simulink model "Gesamtsystem_Prototyp25_01_3"  (R2021b)
settings: Solver=FixedStepDiscrete  StartTime=0.0  StopTime=Inf  RelTol=1e-3  EnableMultiTasking=on
undefined symbols (not defined in the file): Down, GPTRIP1SEL, GPTRIP2SEL, magnitude, TZ1, TZ2, Up
libraries: c2837xDlib x18, hdlsllib x10, simulink x5, c2802xlib x5, c280xlib x3, dspsigops x3, commsequence2 x2, idelinklib_common x2, mcbcontrolslib x2, c2000lib x1, dspstat3 x1
(part 2 of 3)

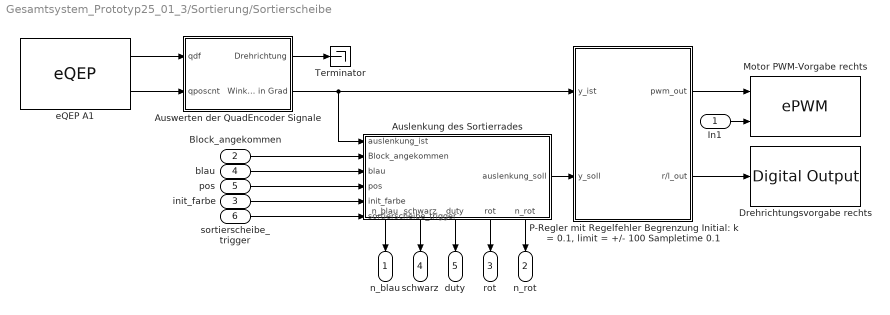
== system Gesamtsystem_Prototyp25_01_3/Sortierung/Sortierscheibe ==
  In1 : Inport
  Block_angekommen : Inport  Port=2
  init_farbe : Inport  Port=3
  blau : Inport  Port=4
  pos : Inport  Port=5
  sortierscheibe_trigger : Inport  Port=6
  Auslenkung des Sortierrades : Stateflow chart  TreatAsAtomicUnit=on
      settings: PortSchema="{\"entries\":[{\"content\":{\"sides\":[{\"content\":{\"connectorIds\":[\"In3\",\"In2\",\"In4\",\"In5\",\"In6\",\"In1\"]},\"type\":\"ConnectorPlacement.EquallySpacedRectSide\",\"uuid\":\"50e19062-f064-4bab-8c9d-33b65ef4a937\"},{\"content\":{\"connectorIds\":[\"Out5\"],\"side\":\"RIGHT\"},\"type\":\"ConnectorPlacement.EquallySpacedRectSide\",\"uuid\":\"30a7e15c-c340-43b9-b3db-9e571d923d3f\"},{\"content\":{\"connectorIds\":[],\"side\":\"TOP\"},\"type\":\"ConnectorPlacement.EquallySpacedRectSide\",\"uuid\":\"40fbcefe-2254-4087-9ee2-3aa6f0d07988\"},{\"content\":{\"connectorIds\":[\"Out4\",\"Out6\",\"Out2\",\"Out3\",\"Out1\"],\"side\":\"BOTTOM\"},\"type\":\"ConnectorPlacement.EquallySpacedRectSide\",\"uuid\":\"44f37ab7-e4d3-4b33-8443-86555161b992\"}]},\"type\":\"ConnectorPlacement.EquallySpacedConnector\",\"uuid\":\"9a2bc586-2b2b-4dda-85c2-1e199ea03007\"}],\"packageUris\":[\"http://schema.mathworks.com/mf0/Connector/R2020b\"],\"version\":\"1.0\"}"
  Auswerten der QuadEncoder Signale : Subsystem
  Drehrichtungsvorgabe rechts : c2837xDlib/Digital Output  GPIO_Number=GPIO88~GPIO95  GPIO_Bit0=off  GPIO_BIT0_Toggle=off  GPIO_Bit1=off  GPIO_BIT1_Toggle=off  GPIO_Bit2=off  GPIO_BIT2_Toggle=off  GPIO_Bit3=off  GPIO_BIT3_Toggle=off  GPIO_Bit4=off  GPIO_BIT4_Toggle=off  GPIO_Bit5=off  GPIO_BIT5_Toggle=off  GPIO_Bit6=on  GPIO_BIT6_Toggle=off  GPIO_Bit7=off  GPIO_BIT7_Toggle=off
      settings: SourceProductBaseCode=TIC2000
  Motor PWM-Vorgabe rechts : c2802xlib/ePWM  PwmType=C2000_Type4  useModule=ePWM6  ePWMxLINKTBPRD=Not Linked  periodUnits=Clock cycles  timerSource=Specify via dialog  timerPeriod_clk=64000  timerPeriod_sec=0.0001  tbshadow=Counter equals to zero  countingMode=Up-Down  phaseActiveEnable=Disable  phaseDirection=Count down after sync  phaseActive=0  synchronizationEnable=off  dcaevt1Sync=off  dcbevt1Sync=off  synchronizationOption=Disable  perSynchronizationOption=Counter equals to period (CTR=PRD)  clockPrescale=1  HSclockPrescale=1  enswap=off  ePWMxAStatus=on  ePWMxAactionLogic1=Set  ePWMxAactionLogic2=Clear  ePWMxAactionLogic3=Clear  ePWMxAactionLogic4=Set  ePWMxAactionLogic5=Do nothing  ePWMxAactionLogic6=Do nothing  ePWMxACSFenable=off  ePWMxACSFvalue=Forcing disable  ePWMxASFreload=Zero  ePWMxBStatus=on  ePWMxBactionLogic1=Set  ePWMxBactionLogic2=Clear  ePWMxBactionLogic3=Do nothing  ePWMxBactionLogic4=Do nothing  ePWMxBactionLogic5=Clear  ePWMxBactionLogic6=Set  ePWMxBCSFenable=off  ePWMxBCSFvalue=Forcing disable  ePWMxBSFreload=Zero  ePWNxBOutWay=off  ePWMxLINKCMPA=Not Linked  CMPAUnits=Percentages  CMPASource=Input port  CMPAValue_per=50  CMPAValue_clk=32000  enCMPAshadow=Counter equals to zero (CTR=Zero)  ePWMxLINKCMPB=Not Linked  CMPBUnits=Percentages  CMPBSource=Input port  CMPBValue_per=25  CMPBValue_clk=32000  enCMPBshadow=Counter equals to zero (CTR=Zero)  ePWMxLINKCMPC=Not Linked  CMPCUnits=Clock cycles  CMPCSource=Specify via dialog  CMPCValue_per=50  CMPCValue_clk=32000  enCMPCshadow=Counter equals to zero (CTR=Zero)  ePWMxLINKCMPD=Not Linked  CMPDUnits=Clock cycles  CMPDSource=Specify via dialog  CMPDValue_per=50  CMPDValue_clk=32000  enCMPDshadow=Counter equals to zero (CTR=Zero)  enableDBePWMxA=off  enableDBePWMxB=off  enhalfcycle=off  DBpolarity=Active high (AH)  DBedgeDelay=Positive  DBSource_ePWMxA=ePWMxA  DBSource_ePWMxB=ePWMxA  DBPeriodUnits=Clock cycles  DBperiodSource=Specify via dialog  REDperiod=0  FEDperiod=0  REDperiod_sec=0  FEDperiod_sec=0  LoadModeDBRED=Immediate without using shadow  LoadModeDBFED=Immediate without using shadow  adcstartModuleA=off  adcrequestEventA=First event  adcstartEventA=Digital Compare Module A Event 1 start of conversion (DCAEVT1.soc)  adcstartEventA_type2=Digital Compare Module A Event 1 start of conversion (DCAEVT1.soc)  adcstartModuleB=off  adcrequestEventB=First event  adcstartEventB=Counter equals to zero (CTR=Zero)  adcstartEventB_type2=Counter equals to zero (CTR=Zero)  intEn=off  intPrd=First event  intSel=Counter equals to zero (CTR=Zero)  intSel_type2=Counter equals to zero (CTR=Zero)  hrpe=off  enHRPWM=off  HRPWM_LoadMode=Counter equals to period (CTR=PRD)  HRPWM_CTLMode=Duty or Period control mode  HRPWM_EDGMode=Both edge  hrpeb=off  enHRPWMB=off  HRPWM_LoadModeB=Counter equals to zero (CTR=ZERO)  HRPWM_CTLModeB=Duty or Period control mode  HRPWM_EDGModeB=Both edge  enHRDBRED=off  enHRDBFED=off  enSFO=on  enautoconv=on  chopperEnable=off  chopperFrequency=1  chopperFirstwidth=1  chopperDuty=12.5%  tripZonesource=Specify via dialog  tzselOSHT1=off  tzselOSHT2=off  tzselOSHT3=off  tzselOSHDCAEV1=off  tzselOSHDCBEV1=off  tzselCBC1=off  tzselCBC2=off  tzselCBC3=off  tzselCBCDCAEV2=off  tzselCBCDCBEV2=off  tzselOSHT4=off  tzselOSHT5=off  tzselOSHT6=off  tzselCBC4=off  tzselCBC5=off  tzselCBC6=off  enTzOstIntr=off  enTzCbcIntr=off  enTzDCAEVT1Intr=off  enTzDCAEVT2Intr=off  enTzDCBEVT1Intr=off  enTzDCBEVT2Intr=off  ePWMxAforced=No action  ePWMxBforced=No action  DCAEVT1forced=No action  DCBEVT1forced=No action  DCAEVT2forced=No action  DCBEVT2forced=No action  dcah=Trip Zone 1 input (TZ1)  dcal=Trip Zone 2 input (TZ2)  dcbh=Trip Zone 1 input (TZ1)  dcbl=Trip Zone 2 input (TZ2)  dcah_type2=GPTRIP1SEL/(TZ1)  dcal_type2=GPTRIP2SEL/(TZ2)  dcbh_type2=GPTRIP1SEL/(TZ1)  dcbl_type2=GPTRIP2SEL/(TZ2)  gendcaevt1=Event disabled  gendcaevt2=Event disabled  gendcbevt1=Event disabled  gendcbevt2=Event disabled  dcaevt1src=DCAEVT1 with sync  dcaevt2src=DCAEVT2 with sync  dcbevt1src=DCBEVT1 with sync  dcbevt2src=DCBEVT2 with sync  pulsesel=Counter equals to zero (CTR=Zero)  blankinv=off  blankoffset=0  blankwidth=0  evsrcsel=Filtered version of DCAEVT1 (DCAEVT1FILT)  encape=off
  "P-Regler mit Regelfehler Begrenzung Initial: k = 0.1, limit = +/- 100 Sampletime 0.1" : Subsystem
  Terminator : Terminator
  eQEP A1 : c280xlib/eQEP  useModule=eQEP1  pcInputmode=Quadrature-count  externalClockrate=2x resolution: Count the rising/falling edge  swapPolarityselection=Clockwise  qdfOutputport=on  qapPolarityselection=off  qbpPolarityselection=off  qipPolarityselection=off  qspPolarityselection=off  igatePolarityselection=off  sampleTime=0.01  pcOutputport=on  pcMaximumvalue=4294967295  indexInitializationcheck=off  indexInitializationevent=Rising edge  strobeInitializationcheck=off  strobeInitializationevent=Rising edge  softwareInitializationcheck=off  softwareInitializationsource=Set to init value at start up  softwareInitializationmode=on  pcInitialvalue=2147483648  pcResetmode=Reset on an index event  ieloutputport=off  indexEventlatch=Rising edge  seloutputport=off  strobeEventlatch=Rising edge  pcefOutputport=off  enableEqepcapture=off  qctmrOutputport=off  qcprdOutputport=off  captureTimerprescaler=128  upEventprescaler=128  overflowErrorflag=off  directionErrorflag=off  captureTimerposition=On position counter read  unitTimerperiod=100000000  captureTimerlatch=off  capturePeriodlatch=off  positionCounterlatch=off  soenPolarityselection=off  spselPolarityselection=Index pin is used for sync output  compareValuesource=Specify via dialog  shadowMode=Load on QPOSCNT=0  compareValue=4294967295  syncOutputwidth=1  polaritySyncoutput=Active high  watchdogEnable=off  watchdogTimer=65535  outport1Datatype=auto  outport2Datatype=auto  outport3Datatype=auto  outport4Datatype=auto  outport5Datatype=auto  outport6Datatype=auto  outport7Datatype=auto  outport8Datatype=auto  outport9Datatype=auto  outport10Datatype=auto  outport11Datatype=auto  outport12Datatype=auto  eqepinterrupt_pce=off  eqepinterrupt_qpe=off  eqepinterrupt_qdc=off  eqepinterrupt_wto=off  eqepinterrupt_pcu=off  eqepinterrupt_pco=off  eqepinterrupt_pcr=off  eqepinterrupt_pcm=off  eqepinterrupt_sel=off  eqepinterrupt_iel=off  eqepinterrupt_uto=off  pheOutputport=off  watchdogOutputport=off  outport13Datatype=auto  outport14Datatype=auto
      settings: SourceProductBaseCode=TIC2000
  n_blau : Outport
  n_rot : Outport  Port=2
  rot : Outport  Port=3
  schwarz : Outport  Port=4
  duty : Outport  Port=5
  wires:
  In1/1 -> Motor PWM-Vorgabe rechts/2
  eQEP A1/1 -> Auswerten der QuadEncoder Signale/1(qdf)
  Auslenkung des Sortierrades/5(auslenkung_soll) -> "P-Regler mit Regelfehler Begrenzung Initial: k = 0.1, limit = +/- 100 Sampletime 0.1"/2(y_soll)
  "P-Regler mit Regelfehler Begrenzung Initial: k = 0.1, limit = +/- 100 Sampletime 0.1"/2(r/l_out) -> Drehrichtungsvorgabe rechts/1
  "P-Regler mit Regelfehler Begrenzung Initial: k = 0.1, limit = +/- 100 Sampletime 0.1"/1(pwm_out) -> Motor PWM-Vorgabe rechts/1
  Auswerten der QuadEncoder Signale/2(Winkel in Grad) -> Auslenkung des Sortierrades/3(auslenkung_ist), "P-Regler mit Regelfehler Begrenzung Initial: k = 0.1, limit = +/- 100 Sampletime 0.1"/1(y_ist)
  eQEP A1/2 -> Auswerten der QuadEncoder Signale/2(qposcnt)
  blau/1 -> Auslenkung des Sortierrades/4(blau)
  Block_angekommen/1 -> Auslenkung des Sortierrades/2(Block_angekommen)
  pos/1 -> Auslenkung des Sortierrades/5(pos)
  Auswerten der QuadEncoder Signale/1(Drehrichtung) -> Terminator/1
  Auslenkung des Sortierrades/1(n_rot) -> n_rot/1
  Auslenkung des Sortierrades/4(n_blau) -> n_blau/1
  Auslenkung des Sortierrades/3(rot) -> rot/1
  Auslenkung des Sortierrades/6(schwarz) -> schwarz/1
  Auslenkung des Sortierrades/2(duty) -> duty/1
  init_farbe/1 -> Auslenkung des Sortierrades/6(init_farbe)
  sortierscheibe_trigger/1 -> Auslenkung des Sortierrades/1(sortierscheibe_trigger)

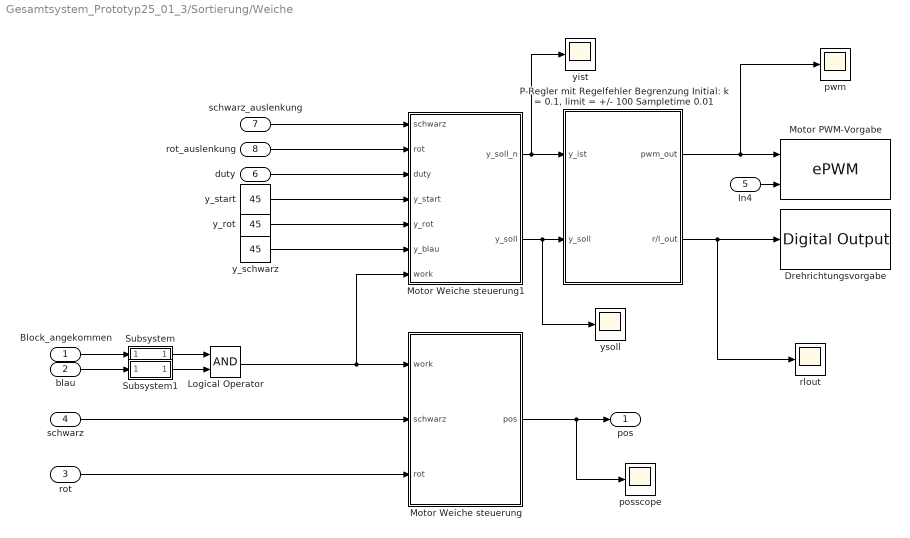
== system Gesamtsystem_Prototyp25_01_3/Sortierung/Weiche ==
  Block_angekommen : Inport
  blau : Inport  Port=2
  rot : Inport  Port=3
  schwarz : Inport  Port=4
  In4 : Inport  Port=5
  duty : Inport  Port=6
  schwarz_auslenkung : Inport  Port=7
  rot_auslenkung : Inport  Port=8
  Drehrichtungsvorgabe : c2837xDlib/Digital Output  GPIO_Number=GPIO120~GPIO127  GPIO_Bit0=off  GPIO_BIT0_Toggle=off  GPIO_Bit1=off  GPIO_BIT1_Toggle=off  GPIO_Bit2=off  GPIO_BIT2_Toggle=off  GPIO_Bit3=on  GPIO_BIT3_Toggle=off  GPIO_Bit4=off  GPIO_BIT4_Toggle=off  GPIO_Bit5=off  GPIO_BIT5_Toggle=off  GPIO_Bit6=off  GPIO_BIT6_Toggle=off  GPIO_Bit7=off  GPIO_BIT7_Toggle=off
      settings: SourceProductBaseCode=TIC2000
  Logical Operator : Logic  AllPortsSameDT=off  OutDataTypeStr=boolean
  Motor PWM-Vorgabe : c2802xlib/ePWM  PwmType=C2000_Type4  useModule=ePWM1  ePWMxLINKTBPRD=Not Linked  periodUnits=Clock cycles  timerSource=Specify via dialog  timerPeriod_clk=64000  timerPeriod_sec=0.0001  tbshadow=Counter equals to zero  countingMode=Up-Down  phaseActiveEnable=Disable  phaseDirection=Count down after sync  phaseActive=0  synchronizationEnable=off  dcaevt1Sync=off  dcbevt1Sync=off  synchronizationOption=Disable  perSynchronizationOption=Counter equals to period (CTR=PRD)  clockPrescale=1  HSclockPrescale=1  enswap=off  ePWMxAStatus=on  ePWMxAactionLogic1=Set  ePWMxAactionLogic2=Clear  ePWMxAactionLogic3=Clear  ePWMxAactionLogic4=Set  ePWMxAactionLogic5=Do nothing  ePWMxAactionLogic6=Do nothing  ePWMxACSFenable=off  ePWMxACSFvalue=Forcing disable  ePWMxASFreload=Zero  ePWMxBStatus=on  ePWMxBactionLogic1=Set  ePWMxBactionLogic2=Clear  ePWMxBactionLogic3=Do nothing  ePWMxBactionLogic4=Do nothing  ePWMxBactionLogic5=Clear  ePWMxBactionLogic6=Set  ePWMxBCSFenable=off  ePWMxBCSFvalue=Forcing disable  ePWMxBSFreload=Zero  ePWNxBOutWay=off  ePWMxLINKCMPA=Not Linked  CMPAUnits=Percentages  CMPASource=Input port  CMPAValue_per=50  CMPAValue_clk=32000  enCMPAshadow=Counter equals to zero (CTR=Zero)  ePWMxLINKCMPB=Not Linked  CMPBUnits=Percentages  CMPBSource=Input port  CMPBValue_per=25  CMPBValue_clk=32000  enCMPBshadow=Counter equals to zero (CTR=Zero)  ePWMxLINKCMPC=Not Linked  CMPCUnits=Clock cycles  CMPCSource=Specify via dialog  CMPCValue_per=50  CMPCValue_clk=32000  enCMPCshadow=Counter equals to zero (CTR=Zero)  ePWMxLINKCMPD=Not Linked  CMPDUnits=Clock cycles  CMPDSource=Specify via dialog  CMPDValue_per=50  CMPDValue_clk=32000  enCMPDshadow=Counter equals to zero (CTR=Zero)  enableDBePWMxA=off  enableDBePWMxB=off  enhalfcycle=off  DBpolarity=Active high (AH)  DBedgeDelay=Positive  DBSource_ePWMxA=ePWMxA  DBSource_ePWMxB=ePWMxA  DBPeriodUnits=Clock cycles  DBperiodSource=Specify via dialog  REDperiod=0  FEDperiod=0  REDperiod_sec=0  FEDperiod_sec=0  LoadModeDBRED=Immediate without using shadow  LoadModeDBFED=Immediate without using shadow  adcstartModuleA=off  adcrequestEventA=First event  adcstartEventA=Digital Compare Module A Event 1 start of conversion (DCAEVT1.soc)  adcstartEventA_type2=Digital Compare Module A Event 1 start of conversion (DCAEVT1.soc)  adcstartModuleB=off  adcrequestEventB=First event  adcstartEventB=Counter equals to zero (CTR=Zero)  adcstartEventB_type2=Counter equals to zero (CTR=Zero)  intEn=off  intPrd=First event  intSel=Counter equals to zero (CTR=Zero)  intSel_type2=Counter equals to zero (CTR=Zero)  hrpe=off  enHRPWM=off  HRPWM_LoadMode=Counter equals to period (CTR=PRD)  HRPWM_CTLMode=Duty or Period control mode  HRPWM_EDGMode=Both edge  hrpeb=off  enHRPWMB=off  HRPWM_LoadModeB=Counter equals to zero (CTR=ZERO)  HRPWM_CTLModeB=Duty or Period control mode  HRPWM_EDGModeB=Both edge  enHRDBRED=off  enHRDBFED=off  enSFO=on  enautoconv=on  chopperEnable=off  chopperFrequency=1  chopperFirstwidth=1  chopperDuty=12.5%  tripZonesource=Specify via dialog  tzselOSHT1=off  tzselOSHT2=off  tzselOSHT3=off  tzselOSHDCAEV1=off  tzselOSHDCBEV1=off  tzselCBC1=off  tzselCBC2=off  tzselCBC3=off  tzselCBCDCAEV2=off  tzselCBCDCBEV2=off  tzselOSHT4=off  tzselOSHT5=off  tzselOSHT6=off  tzselCBC4=off  tzselCBC5=off  tzselCBC6=off  enTzOstIntr=off  enTzCbcIntr=off  enTzDCAEVT1Intr=off  enTzDCAEVT2Intr=off  enTzDCBEVT1Intr=off  enTzDCBEVT2Intr=off  ePWMxAforced=No action  ePWMxBforced=No action  DCAEVT1forced=No action  DCBEVT1forced=No action  DCAEVT2forced=No action  DCBEVT2forced=No action  dcah=Trip Zone 1 input (TZ1)  dcal=Trip Zone 2 input (TZ2)  dcbh=Trip Zone 1 input (TZ1)  dcbl=Trip Zone 2 input (TZ2)  dcah_type2=GPTRIP1SEL/(TZ1)  dcal_type2=GPTRIP2SEL/(TZ2)  dcbh_type2=GPTRIP1SEL/(TZ1)  dcbl_type2=GPTRIP2SEL/(TZ2)  gendcaevt1=Event disabled  gendcaevt2=Event disabled  gendcbevt1=Event disabled  gendcbevt2=Event disabled  dcaevt1src=DCAEVT1 with sync  dcaevt2src=DCAEVT2 with sync  dcbevt1src=DCBEVT1 with sync  dcbevt2src=DCBEVT2 with sync  pulsesel=Counter equals to zero (CTR=Zero)  blankinv=off  blankoffset=0  blankwidth=0  evsrcsel=Filtered version of DCAEVT1 (DCAEVT1FILT)  encape=off
  Motor Weiche steuerung : Stateflow chart  TreatAsAtomicUnit=on
      settings: PortSchema="{\"entries\":[{\"content\":{\"sides\":[{\"content\":{\"connectorIds\":[\"In3\",\"In2\",\"In1\"]},\"type\":\"ConnectorPlacement.EquallySpacedRectSide\",\"uuid\":\"171d8009-52fc-4483-b4bb-3a0c0e7f0866\"},{\"content\":{\"connectorIds\":[\"Out1\"],\"side\":\"RIGHT\"},\"type\":\"ConnectorPlacement.EquallySpacedRectSide\",\"uuid\":\"a1e5e039-26f6-455c-94ae-620f09ecad1d\"},{\"content\":{\"connectorIds\":[],\"side\":\"TOP\"},\"type\":\"ConnectorPlacement.EquallySpacedRectSide\",\"uuid\":\"92e8292a-84f4-4654-b9a0-01a34f9604a2\"}]},\"type\":\"ConnectorPlacement.EquallySpacedConnector\",\"uuid\":\"f344f6ae-6777-4ef0-95d5-423a355c19db\"}],\"packageUris\":[\"http://schema.mathworks.com/mf0/Connector/R2020b\"],\"version\":\"1.0\"}"
  Motor Weiche steuerung1 : Stateflow chart  TreatAsAtomicUnit=on
      settings: PortSchema="{\"entries\":[{\"content\":{\"sides\":[{\"content\":{\"connectorIds\":[\"In2\",\"In1\",\"In7\",\"In4\",\"In5\",\"In6\",\"In3\"]},\"type\":\"ConnectorPlacement.EquallySpacedRectSide\",\"uuid\":\"171d8009-52fc-4483-b4bb-3a0c0e7f0866\"},{\"content\":{\"connectorIds\":[\"Out1\",\"Out2\"],\"side\":\"RIGHT\"},\"type\":\"ConnectorPlacement.EquallySpacedRectSide\",\"uuid\":\"a1e5e039-26f6-455c-94ae-620f09ecad1d\"},{\"content\":{\"connectorIds\":[],\"side\":\"TOP\"},\"type\":\"ConnectorPlacement.EquallySpacedRectSide\",\"uuid\":\"92e8292a-84f4-4654-b9a0-01a34f9604a2\"}]},\"type\":\"ConnectorPlacement.EquallySpacedConnector\",\"uuid\":\"f344f6ae-6777-4ef0-95d5-423a355c19db\"}],\"packageUris\":[\"http://schema.mathworks.com/mf0/Connector/R2020b\"],\"version\":\"1.0\"}"
  "P-Regler mit Regelfehler Begrenzung Initial: k = 0.1, limit = +/- 100 Sampletime 0.01" : Subsystem
  Subsystem : Subsystem
  Subsystem1 : Subsystem
  posscope : Scope
  pwm : Scope
  rlout : Scope
  y_rot : Constant  Value=45
  y_schwarz : Constant  Value=45
  y_start : Constant  Value=45
  yist : Scope
  ysoll : Scope
  pos : Outport
  wires:
  In4/1 -> Motor PWM-Vorgabe/2
  Subsystem1/1(Out1) -> Logical Operator/2
  Subsystem/1(Out1) -> Logical Operator/1
  Logical Operator/1 -> Motor Weiche steuerung1/3(work), Motor Weiche steuerung/3(work)
  rot/1 -> Motor Weiche steuerung/1(rot)
  Motor Weiche steuerung1/1(y_soll_n) -> "P-Regler mit Regelfehler Begrenzung Initial: k = 0.1, limit = +/- 100 Sampletime 0.01"/1(y_ist), yist/1
  Motor Weiche steuerung1/2(y_soll) -> ysoll/1, "P-Regler mit Regelfehler Begrenzung Initial: k = 0.1, limit = +/- 100 Sampletime 0.01"/2(y_soll)
  Block_angekommen/1 -> Subsystem/1(In1)
  "P-Regler mit Regelfehler Begrenzung Initial: k = 0.1, limit = +/- 100 Sampletime 0.01"/1(pwm_out) -> pwm/1, Motor PWM-Vorgabe/1
  "P-Regler mit Regelfehler Begrenzung Initial: k = 0.1, limit = +/- 100 Sampletime 0.01"/2(r/l_out) -> rlout/1, Drehrichtungsvorgabe/1
  blau/1 -> Subsystem1/1(In1)
  Motor Weiche steuerung/1(pos) -> posscope/1, pos/1
  y_start/1 -> Motor Weiche steuerung1/4(y_start)
  y_rot/1 -> Motor Weiche steuerung1/5(y_rot)
  y_schwarz/1 -> Motor Weiche steuerung1/6(y_blau)
  rot_auslenkung/1 -> Motor Weiche steuerung1/1(rot)
  duty/1 -> Motor Weiche steuerung1/7(duty)
  schwarz_auslenkung/1 -> Motor Weiche steuerung1/2(schwarz)
  schwarz/1 -> Motor Weiche steuerung/2(schwarz)

== system Gesamtsystem_Prototyp25_01_3/Sortierung/trigger initialisierung farbe ==
  Digital Input : c2837xDlib/Digital Input  GPIO_Number=GPIO0~GPIO7  GPIO_Bit0=off  GPIO_Bit1=off  GPIO_Bit2=off  GPIO_Bit3=on  GPIO_Bit4=off  GPIO_Bit5=off  GPIO_Bit6=off  GPIO_Bit7=off  sampleTime=0.1  dataType=auto  GPIO_Bit0_Qualification=Sync to SYSCLKOUT  GPIO_Bit1_Qualification=Sync to SYSCLKOUT  GPIO_Bit2_Qualification=Sync to SYSCLKOUT  GPIO_Bit3_Qualification=Sync to SYSCLKOUT  GPIO_Bit4_Qualification=Sync to SYSCLKOUT  GPIO_Bit5_Qualification=Sync to SYSCLKOUT  GPIO_Bit6_Qualification=Sync to SYSCLKOUT  GPIO_Bit7_Qualification=Sync to SYSCLKOUT  Qualification_Period=-1
      settings: SourceProductBaseCode=TIC2000
  Digital Input1 : c2837xDlib/Digital Input  GPIO_Number=GPIO0~GPIO7  GPIO_Bit0=off  GPIO_Bit1=off  GPIO_Bit2=off  GPIO_Bit3=off  GPIO_Bit4=on  GPIO_Bit5=off  GPIO_Bit6=off  GPIO_Bit7=off  sampleTime=0.1  dataType=auto  GPIO_Bit0_Qualification=Sync to SYSCLKOUT  GPIO_Bit1_Qualification=Sync to SYSCLKOUT  GPIO_Bit2_Qualification=Sync to SYSCLKOUT  GPIO_Bit3_Qualification=Sync to SYSCLKOUT  GPIO_Bit4_Qualification=Sync to SYSCLKOUT  GPIO_Bit5_Qualification=Sync to SYSCLKOUT  GPIO_Bit6_Qualification=Sync to SYSCLKOUT  GPIO_Bit7_Qualification=Sync to SYSCLKOUT  Qualification_Period=-1
      settings: SourceProductBaseCode=TIC2000
  Logical Operator : Logic  AllPortsSameDT=off  OutDataTypeStr=boolean
  trigger1 : Outport
  trigger2 : Outport  Port=2
  trigger3 : Outport  Port=3
  wires:
  Digital Input1/1 -> trigger3/1, Logical Operator/2
  Logical Operator/1 -> trigger2/1
  Digital Input/1 -> trigger1/1, Logical Operator/1

== system Gesamtsystem_Prototyp25_01_3/Kommunikation/I2C Receiver/Datastream to bytestream ==
  Datastream : Inport
  Bit Shift1 : hdlsllib/Logic and Bit Operations/Bit Shift  mode=Shift Right Logical  N=8
  Bit Shift2 : hdlsllib/Logic and Bit Operations/Bit Shift  mode=Shift Left Logical  N=8
  Bit Shift4 : hdlsllib/Logic and Bit Operations/Bit Shift  mode=Shift Right Logical  N=8
  Demux : Demux  Outputs=[7 7]
  Interlacer : commsequence2/Interlacer
      settings: SourceProductBaseCode=CM
  Terminator1 : Terminator
  Bytes : Outport
  wires:
  Interlacer/1 -> Bytes/1
  Demux/1 -> Bit Shift1/1, Bit Shift2/1  "testpointQQ"
  Bit Shift2/1 -> Bit Shift4/1
  Bit Shift4/1 -> Interlacer/1
  Demux/2 -> Terminator1/1
  Bit Shift1/1 -> Interlacer/2
  Datastream/1 -> Demux/1

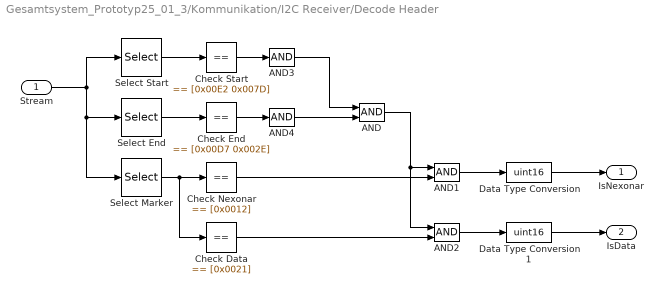
== system Gesamtsystem_Prototyp25_01_3/Kommunikation/I2C Receiver/Decode Header ==
  Stream : Inport
  AND : Logic  IconShape=distinctive  AllPortsSameDT=off  OutDataTypeStr=fixdt(1,16)
  AND1 : Logic  IconShape=distinctive  AllPortsSameDT=off  OutDataTypeStr=fixdt(1,16)
  AND2 : Logic  IconShape=distinctive  AllPortsSameDT=off  OutDataTypeStr=fixdt(1,16)
  AND3 : Logic  Inputs=1  IconShape=distinctive  AllPortsSameDT=off  OutDataTypeStr=fixdt(1,16)
  AND4 : Logic  Inputs=1  IconShape=distinctive  AllPortsSameDT=off  OutDataTypeStr=fixdt(1,16)
  Check Data : simulink/Logic and Bit Operations/Compare To Constant  relop===  const=[0x0021]  OutDataTypeStr=uint8
  Check End : simulink/Logic and Bit Operations/Compare To Constant  relop===  const=[0x00D7 0x002E]  OutDataTypeStr=uint8
  Check Nexonar : simulink/Logic and Bit Operations/Compare To Constant  relop===  const=[0x0012]  OutDataTypeStr=uint8
  Check Start : simulink/Logic and Bit Operations/Compare To Constant  relop===  const=[0x00E2 0x007D]  OutDataTypeStr=uint8
  Data Type Conversion : DataTypeConversion  OutDataTypeStr=uint16
  Data Type Conversion1 : DataTypeConversion  OutDataTypeStr=uint16
  Select End : Selector  InputPortWidth=14  IndexOptions=Index vector (dialog)  Indices=[13 14]  OutputSizes=1
  Select Marker : Selector  InputPortWidth=14  IndexOptions=Index vector (dialog)  Indices=[3]  OutputSizes=1
  Select Start : Selector  InputPortWidth=14  IndexOptions=Index vector (dialog)  Indices=[1 2]  OutputSizes=1
  IsNexonar : Outport
  IsData : Outport  Port=2
  wires:
  Stream/1 -> Select Marker/1, Select End/1, Select Start/1
  Select Start/1 -> Check Start/1
  Select End/1 -> Check End/1
  Select Marker/1 -> Check Data/1, Check Nexonar/1
  Check Nexonar/1 -> AND1/2
  Check Data/1 -> AND2/2
  AND/1 -> AND2/1, AND1/1
  Check Start/1 -> AND3/1
  Check End/1 -> AND4/1
  AND3/1 -> AND/1
  AND4/1 -> AND/2
  AND2/1 -> Data Type Conversion1/1
  Data Type Conversion1/1 -> IsData/1
  AND1/1 -> Data Type Conversion/1
  Data Type Conversion/1 -> IsNexonar/1

== system Gesamtsystem_Prototyp25_01_3/Kommunikation/I2C Receiver/DecodeData ==
  Stream : Inport
  Enable : EnablePort
  Demux : Demux  Outputs=[4 8 2]
  Terminator : Terminator
  Terminator1 : Terminator
  Data : Outport
  wires:
  Stream/1 -> Demux/1
  Demux/2 -> Data/1
  Demux/1 -> Terminator/1
  Demux/3 -> Terminator1/1

== system Gesamtsystem_Prototyp25_01_3/Kommunikation/I2C Receiver/DecodeNexonar ==
  Stream : Inport
  Enable : EnablePort
  Demux : Demux  Outputs=[4 8 2]
  Demux1 : Demux  Outputs=[2 2 2 2]
  Mux : Mux
  Subsystem : Subsystem
  Subsystem1 : Subsystem
  Subsystem2 : Subsystem
  Subsystem3 : Subsystem
  Terminator : Terminator
  Terminator1 : Terminator
  Nexonar : Outport
  wires:
  Stream/1 -> Demux/1
  Demux/3 -> Terminator1/1
  Demux/1 -> Terminator/1
  Demux/2 -> Demux1/1
  Demux1/1 -> Subsystem/1(packed)
  Demux1/2 -> Subsystem1/1(packed)
  Demux1/3 -> Subsystem2/1(packed)
  Demux1/4 -> Subsystem3/1(packed)
  Subsystem/1(unpacked) -> Mux/1  "x"
  Subsystem1/1(unpacked) -> Mux/2  "y"
  Subsystem2/1(unpacked) -> Mux/3  "a"
  Subsystem3/1(unpacked) -> Mux/4  "z"
  Mux/1 -> Nexonar/1  "Nexonar"

== system Gesamtsystem_Prototyp25_01_3/Kommunikation/I2C Reset (behebt Stabilitätsprobleme der I2C-Verbindung)/I2C Reinitialisierung ==
  Trigger : TriggerPort  TriggerType=falling  VariantControl=(inherit)
  I2C Reinitialisierung : MATLAB Function  TreatAsAtomicUnit=on

== system Gesamtsystem_Prototyp25_01_3/Kommunikation/I2C Reset (behebt Stabilitätsprobleme der I2C-Verbindung)/I2C Reset ==
  Trigger : TriggerPort  VariantControl=(inherit)
  I2C Reset : MATLAB Function  TreatAsAtomicUnit=on

== system Gesamtsystem_Prototyp25_01_3/Kommunikation/I2C Transmitter/Subsystem ==
  In1 : Inport
  Enable : EnablePort
  Send WiFi Setup : c280xlib/I2C Transmit  selectModule=I2C_A  addrFormat=7-Bit addressing  saSource=Specify via dialog  SAR=80  bitCount=8  STP=off  RM=off  STR=on
      settings: SourceProductName=Embedded Coder Support Package for Texas Instruments C2000 Processors
  Out1 : Outport
  wires:
  Send WiFi Setup/1 -> Out1/1
  In1/1 -> Send WiFi Setup/1

== system Gesamtsystem_Prototyp25_01_3/Kommunikation/Pack Data Message/Pack Data Bytes ==
  in : Inport
  Bit Shift : hdlsllib/Logic and Bit Operations/Bit Shift  mode=Shift Left Logical  N=8
  Bit Shift1 : hdlsllib/Logic and Bit Operations/Bit Shift  mode=Shift Right Logical  N=8
  Data Type Conversion : DataTypeConversion  OutDataTypeStr=uint16
  Pad1 : dspsigops/Pad  padAlong=Columns  dimsToPad=1  valSrc=Specify via dialog  padVal=255  spec=Output size  padNumOutRowsSpecMethod=User-specified  numOutRows=8  padNumOutColsSpecMethod=User-specified  numOutCols=1  isVarDimsMode=off  padBeginning=0  padEnd=0  outSizeMode=User-specified  outSize=1  padSigAt=End  trunc_flag=None  roundingMode=Floor  overflowMode=off  truncOrWrapMode=Truncate  wrap_flag=None
      settings: SourceProductBaseCode=DS
  out : Outport
  wires:
  Pad1/1 -> Bit Shift/1
  Data Type Conversion/1 -> Pad1/1
  Bit Shift1/1 -> out/1
  Bit Shift/1 -> Bit Shift1/1
  in/1 -> Data Type Conversion/1

== system Gesamtsystem_Prototyp25_01_3/Navigation und Uebergabe/Abwurf und Uebergabe/P-Regler mit Regelfehler Begrenzung Initial: k = 0.1, limit = +//- 100 Sampletime 0.1 ==
  y_soll_rb : Inport
  y_ist : Inport  Port=2
  Abs : Abs  SampleTime=0.01
  Begrenzung : Saturate  UpperLimit=80  LowerLimit=0
  Betrag : MATLAB Function  TreatAsAtomicUnit=on  SystemSampleTime=0.01
  Dead Zone : DeadZone  LowerValue=-5  UpperValue=5  SaturateOnIntegerOverflow=on
  Richtung : MATLAB Function  TreatAsAtomicUnit=on  SystemSampleTime=0.01
  Sum : Sum  Inputs=|-+  SampleTime=0.01
  Verstaerkung : Gain  SampleTime=0.01
  pwm_out : Outport  VectorParamsAs1DForOutWhenUnconnected=off
  r/l_out : Outport  Port=2  VectorParamsAs1DForOutWhenUnconnected=off
  wires:
  Betrag/1(y) -> pwm_out/1
  Verstaerkung/1 -> Abs/1, Richtung/1(u)
  Sum/1 -> Dead Zone/1
  Abs/1 -> Begrenzung/1
  y_soll_rb/1 -> Sum/2
  Richtung/1(y) -> r/l_out/1
  y_ist/1 -> Sum/1
  Begrenzung/1 -> Betrag/1(u)
  Dead Zone/1 -> Verstaerkung/1

== system Gesamtsystem_Prototyp25_01_3/Navigation und Uebergabe/Abwurf und Uebergabe/P-Regler mit Regelfehler Begrenzung Initial: k = 0.1, limit = +//- 100 Sampletime 0.2 ==
  y_soll_s : Inport
  y_ist : Inport  Port=2
  Abs : Abs  SampleTime=0.01
  Begrenzung : Saturate  UpperLimit=80  LowerLimit=0
  Betrag : MATLAB Function  TreatAsAtomicUnit=on  SystemSampleTime=0.01
  Dead Zone : DeadZone  LowerValue=-5  UpperValue=5  SaturateOnIntegerOverflow=on
  Richtung : MATLAB Function  TreatAsAtomicUnit=on  SystemSampleTime=0.01
  Sum : Sum  Inputs=|-+  SampleTime=0.01
  Verstaerkung : Gain  Gain=5  SampleTime=0.01
  pwm_out : Outport  VectorParamsAs1DForOutWhenUnconnected=off
  r/l_out : Outport  Port=2  VectorParamsAs1DForOutWhenUnconnected=off
  wires:
  Betrag/1(y) -> pwm_out/1
  Verstaerkung/1 -> Abs/1, Richtung/1(u)
  Sum/1 -> Dead Zone/1
  Abs/1 -> Begrenzung/1
  y_soll_s/1 -> Sum/2
  Richtung/1(y) -> r/l_out/1
  y_ist/1 -> Sum/1
  Begrenzung/1 -> Betrag/1(u)
  Dead Zone/1 -> Verstaerkung/1

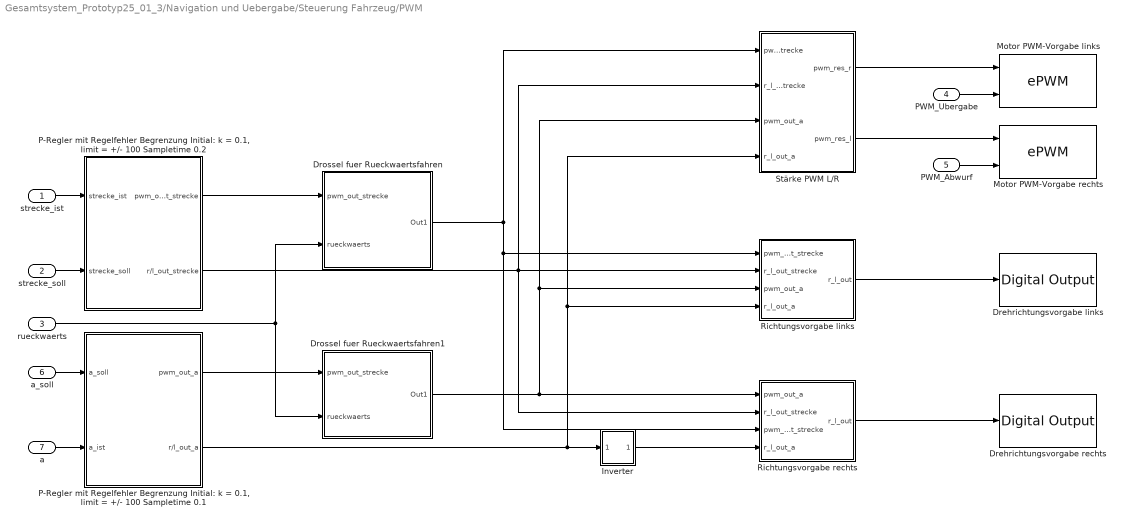
== system Gesamtsystem_Prototyp25_01_3/Navigation und Uebergabe/Steuerung Fahrzeug/PWM ==
  strecke_ist : Inport
  strecke_soll : Inport  Port=2
  rueckwaerts : Inport  Port=3
  PWM_Ubergabe : Inport  Port=4
  PWM_Abwurf : Inport  Port=5
  a_soll : Inport  Port=6
  a : Inport  Port=7
  Drehrichtungsvorgabe links : c2837xDlib/Digital Output  GPIO_Number=GPIO128~GPIO135  GPIO_Bit0=off  GPIO_BIT0_Toggle=off  GPIO_Bit1=off  GPIO_BIT1_Toggle=off  GPIO_Bit2=off  GPIO_BIT2_Toggle=off  GPIO_Bit3=on  GPIO_BIT3_Toggle=off  GPIO_Bit4=off  GPIO_BIT4_Toggle=off  GPIO_Bit5=off  GPIO_BIT5_Toggle=off  GPIO_Bit6=off  GPIO_BIT6_Toggle=off  GPIO_Bit7=off  GPIO_BIT7_Toggle=off
      settings: SourceProductBaseCode=TIC2000
  Drehrichtungsvorgabe rechts : c2837xDlib/Digital Output  GPIO_Number=GPIO128~GPIO135  GPIO_Bit0=off  GPIO_BIT0_Toggle=off  GPIO_Bit1=off  GPIO_BIT1_Toggle=off  GPIO_Bit2=on  GPIO_BIT2_Toggle=off  GPIO_Bit3=off  GPIO_BIT3_Toggle=off  GPIO_Bit4=off  GPIO_BIT4_Toggle=off  GPIO_Bit5=off  GPIO_BIT5_Toggle=off  GPIO_Bit6=off  GPIO_BIT6_Toggle=off  GPIO_Bit7=off  GPIO_BIT7_Toggle=off
      settings: SourceProductBaseCode=TIC2000
  Drossel fuer Rueckwaertsfahren : Subsystem
  Drossel fuer Rueckwaertsfahren1 : Subsystem
  Inverter : Subsystem
  Motor PWM-Vorgabe links : c2802xlib/ePWM  PwmType=C2000_Type4  useModule=ePWM4  ePWMxLINKTBPRD=Not Linked  periodUnits=Clock cycles  timerSource=Specify via dialog  timerPeriod_clk=64000  timerPeriod_sec=0.0001  tbshadow=Counter equals to zero  countingMode=Up-Down  phaseActiveEnable=Disable  phaseDirection=Count down after sync  phaseActive=0  synchronizationEnable=off  dcaevt1Sync=off  dcbevt1Sync=off  synchronizationOption=Disable  perSynchronizationOption=Counter is incrementing and equals to the compare C register (CTRU=CMPC)  clockPrescale=1  HSclockPrescale=1  enswap=off  ePWMxAStatus=on  ePWMxAactionLogic1=Set  ePWMxAactionLogic2=Clear  ePWMxAactionLogic3=Clear  ePWMxAactionLogic4=Set  ePWMxAactionLogic5=Do nothing  ePWMxAactionLogic6=Do nothing  ePWMxACSFenable=off  ePWMxACSFvalue=Forcing disable  ePWMxASFreload=Zero  ePWMxBStatus=on  ePWMxBactionLogic1=Set  ePWMxBactionLogic2=Clear  ePWMxBactionLogic3=Do nothing  ePWMxBactionLogic4=Do nothing  ePWMxBactionLogic5=Clear  ePWMxBactionLogic6=Set  ePWMxBCSFenable=off  ePWMxBCSFvalue=Forcing disable  ePWMxBSFreload=Zero  ePWNxBOutWay=off  ePWMxLINKCMPA=Not Linked  CMPAUnits=Percentages  CMPASource=Input port  CMPAValue_per=50  CMPAValue_clk=32000  enCMPAshadow=Counter equals to zero (CTR=Zero)  ePWMxLINKCMPB=Not Linked  CMPBUnits=Percentages  CMPBSource=Input port  CMPBValue_per=25  CMPBValue_clk=32000  enCMPBshadow=Counter equals to zero (CTR=Zero)  ePWMxLINKCMPC=Not Linked  CMPCUnits=Clock cycles  CMPCSource=Specify via dialog  CMPCValue_per=50  CMPCValue_clk=32000  enCMPCshadow=Counter equals to zero (CTR=Zero)  ePWMxLINKCMPD=Not Linked  CMPDUnits=Clock cycles  CMPDSource=Specify via dialog  CMPDValue_per=50  CMPDValue_clk=32000  enCMPDshadow=Counter equals to zero (CTR=Zero)  enableDBePWMxA=off  enableDBePWMxB=off  enhalfcycle=off  DBpolarity=Active high (AH)  DBedgeDelay=Positive  DBSource_ePWMxA=ePWMxA  DBSource_ePWMxB=ePWMxA  DBPeriodUnits=Clock cycles  DBperiodSource=Specify via dialog  REDperiod=0  FEDperiod=0  REDperiod_sec=0  FEDperiod_sec=0  LoadModeDBRED=Immediate without using shadow  LoadModeDBFED=Immediate without using shadow  adcstartModuleA=off  adcrequestEventA=First event  adcstartEventA=Digital Compare Module A Event 1 start of conversion (DCAEVT1.soc)  adcstartEventA_type2=Digital Compare Module A Event 1 start of conversion (DCAEVT1.soc)  adcstartModuleB=off  adcrequestEventB=First event  adcstartEventB=Counter equals to zero (CTR=Zero)  adcstartEventB_type2=Counter equals to zero (CTR=Zero)  intEn=off  intPrd=First event  intSel=Counter equals to zero (CTR=Zero)  intSel_type2=Counter equals to zero (CTR=Zero)  hrpe=off  enHRPWM=off  HRPWM_LoadMode=Counter equals to period (CTR=PRD)  HRPWM_CTLMode=Duty or Period control mode  HRPWM_EDGMode=Both edge  hrpeb=off  enHRPWMB=off  HRPWM_LoadModeB=Counter equals to zero (CTR=ZERO)  HRPWM_CTLModeB=Duty or Period control mode  HRPWM_EDGModeB=Both edge  enHRDBRED=off  enHRDBFED=off  enSFO=on  enautoconv=on  chopperEnable=off  chopperFrequency=1  chopperFirstwidth=1  chopperDuty=12.5%  tripZonesource=Specify via dialog  tzselOSHT1=off  tzselOSHT2=off  tzselOSHT3=off  tzselOSHDCAEV1=off  tzselOSHDCBEV1=off  tzselCBC1=off  tzselCBC2=off  tzselCBC3=off  tzselCBCDCAEV2=off  tzselCBCDCBEV2=off  tzselOSHT4=off  tzselOSHT5=off  tzselOSHT6=off  tzselCBC4=off  tzselCBC5=off  tzselCBC6=off  enTzOstIntr=off  enTzCbcIntr=off  enTzDCAEVT1Intr=off  enTzDCAEVT2Intr=off  enTzDCBEVT1Intr=off  enTzDCBEVT2Intr=off  ePWMxAforced=No action  ePWMxBforced=No action  DCAEVT1forced=No action  DCBEVT1forced=No action  DCAEVT2forced=No action  DCBEVT2forced=No action  dcah=Trip Zone 1 input (TZ1)  dcal=Trip Zone 2 input (TZ2)  dcbh=Trip Zone 1 input (TZ1)  dcbl=Trip Zone 2 input (TZ2)  dcah_type2=GPTRIP1SEL/(TZ1)  dcal_type2=GPTRIP2SEL/(TZ2)  dcbh_type2=GPTRIP1SEL/(TZ1)  dcbl_type2=GPTRIP2SEL/(TZ2)  gendcaevt1=Event disabled  gendcaevt2=Event disabled  gendcbevt1=Event disabled  gendcbevt2=Event disabled  dcaevt1src=DCAEVT1 with sync  dcaevt2src=DCAEVT2 with sync  dcbevt1src=DCBEVT1 with sync  dcbevt2src=DCBEVT2 with sync  pulsesel=Counter equals to zero (CTR=Zero)  blankinv=off  blankoffset=0  blankwidth=0  evsrcsel=Filtered version of DCAEVT1 (DCAEVT1FILT)  encape=off
  Motor PWM-Vorgabe rechts : c2802xlib/ePWM  PwmType=C2000_Type4  useModule=ePWM5  ePWMxLINKTBPRD=Not Linked  periodUnits=Clock cycles  timerSource=Specify via dialog  timerPeriod_clk=64000  timerPeriod_sec=0.0001  tbshadow=Counter equals to zero  countingMode=Up-Down  phaseActiveEnable=Disable  phaseDirection=Count down after sync  phaseActive=0  synchronizationEnable=off  dcaevt1Sync=off  dcbevt1Sync=off  synchronizationOption=Disable  perSynchronizationOption=Counter equals to period (CTR=PRD)  clockPrescale=1  HSclockPrescale=1  enswap=off  ePWMxAStatus=on  ePWMxAactionLogic1=Set  ePWMxAactionLogic2=Clear  ePWMxAactionLogic3=Clear  ePWMxAactionLogic4=Set  ePWMxAactionLogic5=Do nothing  ePWMxAactionLogic6=Do nothing  ePWMxACSFenable=off  ePWMxACSFvalue=Forcing disable  ePWMxASFreload=Zero  ePWMxBStatus=on  ePWMxBactionLogic1=Set  ePWMxBactionLogic2=Clear  ePWMxBactionLogic3=Do nothing  ePWMxBactionLogic4=Do nothing  ePWMxBactionLogic5=Clear  ePWMxBactionLogic6=Set  ePWMxBCSFenable=off  ePWMxBCSFvalue=Forcing disable  ePWMxBSFreload=Zero  ePWNxBOutWay=off  ePWMxLINKCMPA=Not Linked  CMPAUnits=Percentages  CMPASource=Input port  CMPAValue_per=50  CMPAValue_clk=32000  enCMPAshadow=Counter equals to zero (CTR=Zero)  ePWMxLINKCMPB=Not Linked  CMPBUnits=Percentages  CMPBSource=Input port  CMPBValue_per=25  CMPBValue_clk=32000  enCMPBshadow=Counter equals to zero (CTR=Zero)  ePWMxLINKCMPC=Not Linked  CMPCUnits=Clock cycles  CMPCSource=Specify via dialog  CMPCValue_per=50  CMPCValue_clk=32000  enCMPCshadow=Counter equals to zero (CTR=Zero)  ePWMxLINKCMPD=Not Linked  CMPDUnits=Clock cycles  CMPDSource=Specify via dialog  CMPDValue_per=50  CMPDValue_clk=32000  enCMPDshadow=Counter equals to zero (CTR=Zero)  enableDBePWMxA=off  enableDBePWMxB=off  enhalfcycle=off  DBpolarity=Active high (AH)  DBedgeDelay=Positive  DBSource_ePWMxA=ePWMxA  DBSource_ePWMxB=ePWMxA  DBPeriodUnits=Clock cycles  DBperiodSource=Specify via dialog  REDperiod=0  FEDperiod=0  REDperiod_sec=0  FEDperiod_sec=0  LoadModeDBRED=Immediate without using shadow  LoadModeDBFED=Immediate without using shadow  adcstartModuleA=off  adcrequestEventA=First event  adcstartEventA=Digital Compare Module A Event 1 start of conversion (DCAEVT1.soc)  adcstartEventA_type2=Digital Compare Module A Event 1 start of conversion (DCAEVT1.soc)  adcstartModuleB=off  adcrequestEventB=First event  adcstartEventB=Counter equals to zero (CTR=Zero)  adcstartEventB_type2=Counter equals to zero (CTR=Zero)  intEn=off  intPrd=First event  intSel=Counter equals to zero (CTR=Zero)  intSel_type2=Counter equals to zero (CTR=Zero)  hrpe=off  enHRPWM=off  HRPWM_LoadMode=Counter equals to period (CTR=PRD)  HRPWM_CTLMode=Duty or Period control mode  HRPWM_EDGMode=Both edge  hrpeb=off  enHRPWMB=off  HRPWM_LoadModeB=Counter equals to zero (CTR=ZERO)  HRPWM_CTLModeB=Duty or Period control mode  HRPWM_EDGModeB=Both edge  enHRDBRED=off  enHRDBFED=off  enSFO=on  enautoconv=on  chopperEnable=off  chopperFrequency=1  chopperFirstwidth=1  chopperDuty=12.5%  tripZonesource=Specify via dialog  tzselOSHT1=off  tzselOSHT2=off  tzselOSHT3=off  tzselOSHDCAEV1=off  tzselOSHDCBEV1=off  tzselCBC1=off  tzselCBC2=off  tzselCBC3=off  tzselCBCDCAEV2=off  tzselCBCDCBEV2=off  tzselOSHT4=off  tzselOSHT5=off  tzselOSHT6=off  tzselCBC4=off  tzselCBC5=off  tzselCBC6=off  enTzOstIntr=off  enTzCbcIntr=off  enTzDCAEVT1Intr=off  enTzDCAEVT2Intr=off  enTzDCBEVT1Intr=off  enTzDCBEVT2Intr=off  ePWMxAforced=No action  ePWMxBforced=No action  DCAEVT1forced=No action  DCBEVT1forced=No action  DCAEVT2forced=No action  DCBEVT2forced=No action  dcah=Trip Zone 1 input (TZ1)  dcal=Trip Zone 2 input (TZ2)  dcbh=Trip Zone 1 input (TZ1)  dcbl=Trip Zone 2 input (TZ2)  dcah_type2=GPTRIP1SEL/(TZ1)  dcal_type2=GPTRIP2SEL/(TZ2)  dcbh_type2=GPTRIP1SEL/(TZ1)  dcbl_type2=GPTRIP2SEL/(TZ2)  gendcaevt1=Event disabled  gendcaevt2=Event disabled  gendcbevt1=Event disabled  gendcbevt2=Event disabled  dcaevt1src=DCAEVT1 with sync  dcaevt2src=DCAEVT2 with sync  dcbevt1src=DCBEVT1 with sync  dcbevt2src=DCBEVT2 with sync  pulsesel=Counter equals to zero (CTR=Zero)  blankinv=off  blankoffset=0  blankwidth=0  evsrcsel=Filtered version of DCAEVT1 (DCAEVT1FILT)  encape=off
  "P-Regler mit Regelfehler Begrenzung Initial: k = 0.1, limit = +/- 100 Sampletime 0.1" : Subsystem
  "P-Regler mit Regelfehler Begrenzung Initial: k = 0.1, limit = +/- 100 Sampletime 0.2" : Subsystem
  Richtungsvorgabe links : Stateflow chart  TreatAsAtomicUnit=on
      settings: PortSchema="{\"entries\":[{\"content\":{\"sides\":[{\"content\":{\"connectorIds\":[\"In3\",\"In1\",\"In4\",\"In2\"]},\"type\":\"ConnectorPlacement.EquallySpacedRectSide\",\"uuid\":\"43ce88f5-1469-497e-a051-ba954b178805\"},{\"content\":{\"connectorIds\":[\"Out1\"],\"side\":\"RIGHT\"},\"type\":\"ConnectorPlacement.EquallySpacedRectSide\",\"uuid\":\"cbcca745-edd0-4de4-9e7f-81e160884945\"},{\"content\":{\"connectorIds\":[],\"side\":\"TOP\"},\"type\":\"ConnectorPlacement.EquallySpacedRectSide\",\"uuid\":\"26990ae6-7e57-4f33-8f48-f3e7ff204d3e\"},{\"content\":{\"connectorIds\":[],\"side\":\"BOTTOM\"},\"type\":\"ConnectorPlacement.EquallySpacedRectSide\",\"uuid\":\"96722544-5cbd-4a59-98ae-816f7f6d82ef\"}]},\"type\":\"ConnectorPlacement.EquallySpacedConnector\",\"uuid\":\"50553682-979e-4462-a950-9c1f22c21ad0\"}],\"packageUris\":[\"http://schema.mathworks.com/mf0/Connector/R2020b\"],\"version\":\"1.0\"}"
  Richtungsvorgabe rechts : Stateflow chart  TreatAsAtomicUnit=on
      settings: PortSchema="{\"entries\":[{\"content\":{\"sides\":[{\"content\":{\"connectorIds\":[\"In4\",\"In1\",\"In3\",\"In2\"]},\"type\":\"ConnectorPlacement.EquallySpacedRectSide\",\"uuid\":\"43ce88f5-1469-497e-a051-ba954b178805\"},{\"content\":{\"connectorIds\":[\"Out1\"],\"side\":\"RIGHT\"},\"type\":\"ConnectorPlacement.EquallySpacedRectSide\",\"uuid\":\"cbcca745-edd0-4de4-9e7f-81e160884945\"},{\"content\":{\"connectorIds\":[],\"side\":\"TOP\"},\"type\":\"ConnectorPlacement.EquallySpacedRectSide\",\"uuid\":\"26990ae6-7e57-4f33-8f48-f3e7ff204d3e\"},{\"content\":{\"connectorIds\":[],\"side\":\"BOTTOM\"},\"type\":\"ConnectorPlacement.EquallySpacedRectSide\",\"uuid\":\"96722544-5cbd-4a59-98ae-816f7f6d82ef\"}]},\"type\":\"ConnectorPlacement.EquallySpacedConnector\",\"uuid\":\"50553682-979e-4462-a950-9c1f22c21ad0\"}],\"packageUris\":[\"http://schema.mathworks.com/mf0/Connector/R2020b\"],\"version\":\"1.0\"}"
  Stärke PWM L/R : Stateflow chart  TreatAsAtomicUnit=on
      settings: PortSchema="{\"entries\":[{\"content\":{\"sides\":[{\"content\":{\"connectorIds\":[\"In3\",\"In2\",\"In4\",\"In1\"]},\"type\":\"ConnectorPlacement.EquallySpacedRectSide\",\"uuid\":\"c076548a-8c40-4c2a-9129-11e36bd922ff\"},{\"content\":{\"connectorIds\":[\"Out2\",\"Out1\"],\"side\":\"RIGHT\"},\"type\":\"ConnectorPlacement.EquallySpacedRectSide\",\"uuid\":\"384b694f-2676-4168-bfa5-0787da96f974\"},{\"content\":{\"connectorIds\":[],\"side\":\"TOP\"},\"type\":\"ConnectorPlacement.EquallySpacedRectSide\",\"uuid\":\"cbe6e1c7-9e75-41b5-b50f-b847b47c03cc\"},{\"content\":{\"connectorIds\":[],\"side\":\"BOTTOM\"},\"type\":\"ConnectorPlacement.EquallySpacedRectSide\",\"uuid\":\"71d6e623-91fe-46b8-bb98-1f03970657ba\"}]},\"type\":\"ConnectorPlacement.EquallySpacedConnector\",\"uuid\":\"e4a06fb8-2f13-4332-9a84-3831f1358431\"}],\"packageUris\":[\"http://schema.mathworks.com/mf0/Connector/R2020b\"],\"version\":\"1.0\"}"
  wires:
  "P-Regler mit Regelfehler Begrenzung Initial: k = 0.1, limit = +/- 100 Sampletime 0.1"/2(r/l_out_a) -> Stärke PWM L/R/1(r_l_out_a), Richtungsvorgabe links/2(r_l_out_a), Inverter/1(In1)
  Drossel fuer Rueckwaertsfahren/1(Out1) -> Stärke PWM L/R/3(pwm_out_strecke), Richtungsvorgabe links/3(pwm_out_strecke), Richtungsvorgabe rechts/3(pwm_out_strecke)
  "P-Regler mit Regelfehler Begrenzung Initial: k = 0.1, limit = +/- 100 Sampletime 0.2"/2(r/l_out_strecke) -> Richtungsvorgabe rechts/1(r_l_out_strecke), Richtungsvorgabe links/1(r_l_out_strecke), Stärke PWM L/R/2(r_l_out_strecke)
  a/1 -> "P-Regler mit Regelfehler Begrenzung Initial: k = 0.1, limit = +/- 100 Sampletime 0.1"/2(a_ist)
  PWM_Ubergabe/1 -> Motor PWM-Vorgabe links/2
  a_soll/1 -> "P-Regler mit Regelfehler Begrenzung Initial: k = 0.1, limit = +/- 100 Sampletime 0.1"/1(a_soll)
  PWM_Abwurf/1 -> Motor PWM-Vorgabe rechts/2
  strecke_ist/1 -> "P-Regler mit Regelfehler Begrenzung Initial: k = 0.1, limit = +/- 100 Sampletime 0.2"/1(strecke_ist)
  Drossel fuer Rueckwaertsfahren1/1(Out1) -> Richtungsvorgabe links/4(pwm_out_a), Stärke PWM L/R/4(pwm_out_a), Richtungsvorgabe rechts/4(pwm_out_a)
  Inverter/1(Out1) -> Richtungsvorgabe rechts/2(r_l_out_a)
  strecke_soll/1 -> "P-Regler mit Regelfehler Begrenzung Initial: k = 0.1, limit = +/- 100 Sampletime 0.2"/2(strecke_soll)
  Stärke PWM L/R/2(pwm_res_r) -> Motor PWM-Vorgabe links/1
  Stärke PWM L/R/1(pwm_res_l) -> Motor PWM-Vorgabe rechts/1
  Richtungsvorgabe links/1(r_l_out) -> Drehrichtungsvorgabe links/1
  Richtungsvorgabe rechts/1(r_l_out) -> Drehrichtungsvorgabe rechts/1
  rueckwaerts/1 -> Drossel fuer Rueckwaertsfahren/2(rueckwaerts), Drossel fuer Rueckwaertsfahren1/2(rueckwaerts)
  "P-Regler mit Regelfehler Begrenzung Initial: k = 0.1, limit = +/- 100 Sampletime 0.2"/1(pwm_out_strecke) -> Drossel fuer Rueckwaertsfahren/1(pwm_out_strecke)
  "P-Regler mit Regelfehler Begrenzung Initial: k = 0.1, limit = +/- 100 Sampletime 0.1"/1(pwm_out_a) -> Drossel fuer Rueckwaertsfahren1/1(pwm_out_strecke)

== system Gesamtsystem_Prototyp25_01_3/Navigation und Uebergabe/Steuerung Fahrzeug/Steuerung oder Rueckwaertsgang ==
  strecke_soll : Inport
  strecke_ist : Inport  Port=2
  rueckwaerts : Inport  Port=3
  Switch1 : Switch  Criteria=u2 > Threshold
  Switch5 : Switch  Criteria=u2 > Threshold
  Out1 : Outport
  Out2 : Outport  Port=2
  wires:
  Switch5/1 -> Out1/1
  rueckwaerts/1 -> Switch5/2, Switch1/2
  strecke_ist/1 -> Switch5/1, Switch1/3
  strecke_soll/1 -> Switch5/3, Switch1/1
  Switch1/1 -> Out2/1

== system Gesamtsystem_Prototyp25_01_3/Navigation und Uebergabe/Steuerung Fahrzeug/Streckenberechnung ==
  x : Inport
  x_soll : Inport  Port=2
  y_soll : Inport  Port=3
  y : Inport  Port=4
  Add : Sum  Inputs=+-
  Add1 : Sum
  Add2 : Sum  Inputs=+-
  Magnitude Squared : Math  Operator=magnitude^2  SaturateOnIntegerOverflow=on
  Magnitude Squared1 : Math  Operator=magnitude^2  SaturateOnIntegerOverflow=on
  Sqrt : Sqrt  SaturateOnIntegerOverflow=on
  strecke_ist : Outport
  wires:
  x_soll/1 -> Add2/2
  Add2/1 -> Magnitude Squared1/1
  y_soll/1 -> Add/2
  Add/1 -> Magnitude Squared/1
  x/1 -> Add2/1
  Magnitude Squared1/1 -> Add1/2
  Magnitude Squared/1 -> Add1/1
  y/1 -> Add/1
  Add1/1 -> Sqrt/1
  Sqrt/1 -> strecke_ist/1

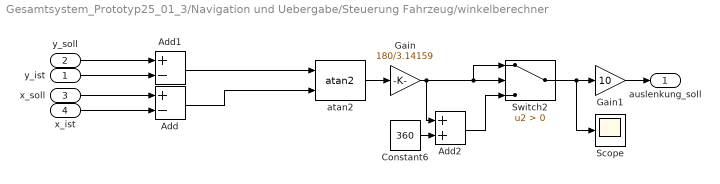
== system Gesamtsystem_Prototyp25_01_3/Navigation und Uebergabe/Steuerung Fahrzeug/winkelberechner ==
  y_ist : Inport
  y_soll : Inport  Port=2
  x_soll : Inport  Port=3
  x_ist : Inport  Port=4
  Add : Sum  Inputs=+-
  Add1 : Sum  Inputs=+-
  Add2 : Sum
  Constant6 : Constant  Value=360
  Gain : Gain  Gain=180/3.14159
  Gain1 : Gain  Gain=10
  Scope : Scope
  Switch2 : Switch  Criteria=u2 > Threshold
  atan2 : mcbcontrolslib/atan2  outputUnit=Radians
      settings: SourceProductBaseCode=MT
  auslenkung_soll : Outport
  wires:
  Gain/1 -> Add2/1, Switch2/1, Switch2/2
  Add/1 -> atan2/2
  atan2/1 -> Gain/1
  Constant6/1 -> Add2/2
  Add2/1 -> Switch2/3
  x_soll/1 -> Add/1
  Add1/1 -> atan2/1
  y_ist/1 -> Add1/2
  y_soll/1 -> Add1/1
  x_ist/1 -> Add/2
  Gain1/1 -> auslenkung_soll/1
  Switch2/1 -> Scope/1, Gain1/1

== system Gesamtsystem_Prototyp25_01_3/Sortierung/Sortierscheibe/Auswerten der QuadEncoder Signale ==
  qdf : Inport
  qposcnt : Inport  Port=2
  Add : Sum  Inputs=+-
  Add1 : Sum  Inputs=+-
  Constant : Constant  Value=2147483647
  Constant1 : Constant  Value=4294967295
  GainMotorShaft2 : Gain  Gain=1/48
  GainOutputShaft2 : Gain  Gain=1/98.78  OutDataTypeStr=double
  RevToDeg2 : Gain  Gain=360
  Switch : Switch  Criteria=u2 > Threshold
  Drehrichtung : Outport
  Winkel in Grad : Outport  Port=2
  wires:
  qdf/1 -> Drehrichtung/1
  qposcnt/1 -> Add1/1, Add/1, Switch/3
  Add/1 -> Switch/2
  Constant/1 -> Add/2
  Constant1/1 -> Add1/2
  Add1/1 -> Switch/1
  GainMotorShaft2/1 -> GainOutputShaft2/1
  RevToDeg2/1 -> GainMotorShaft2/1
  Switch/1 -> RevToDeg2/1
  GainOutputShaft2/1 -> Winkel in Grad/1

== system Gesamtsystem_Prototyp25_01_3/Sortierung/Sortierscheibe/P-Regler mit Regelfehler Begrenzung Initial: k = 0.1, limit = +//- 100 Sampletime 0.1 ==
  y_ist : Inport
  y_soll : Inport  Port=2
  Abs : Abs  SampleTime=0.01
  Begrenzung : Saturate  UpperLimit=80  LowerLimit=3
  Betrag : MATLAB Function  TreatAsAtomicUnit=on  SystemSampleTime=0.01
  Dead Zone : DeadZone  SaturateOnIntegerOverflow=on
  Richtung : MATLAB Function  TreatAsAtomicUnit=on  SystemSampleTime=0.01
  Sum : Sum  Inputs=|-+  SampleTime=0.01
  Verstaerkung : Gain  Gain=2  SampleTime=0.01
  pwm_out : Outport  VectorParamsAs1DForOutWhenUnconnected=off
  r/l_out : Outport  Port=2  VectorParamsAs1DForOutWhenUnconnected=off
  wires:
  Betrag/1(y) -> pwm_out/1
  Verstaerkung/1 -> Abs/1, Richtung/1(u)
  Sum/1 -> Dead Zone/1
  Abs/1 -> Begrenzung/1
  y_soll/1 -> Sum/2
  Richtung/1(y) -> r/l_out/1
  y_ist/1 -> Sum/1
  Begrenzung/1 -> Betrag/1(u)
  Dead Zone/1 -> Verstaerkung/1

== system Gesamtsystem_Prototyp25_01_3/Sortierung/Weiche/P-Regler mit Regelfehler Begrenzung Initial: k = 0.1, limit = +//- 100 Sampletime 0.01 ==
  y_ist : Inport
  y_soll : Inport  Port=2
  Abs : Abs  SampleTime=0.01
  Begrenzung : Saturate  UpperLimit=100  LowerLimit=0
  Betrag : MATLAB Function  TreatAsAtomicUnit=on  SystemSampleTime=0.01
  Dead Zone : DeadZone  LowerValue=-3  UpperValue=3  SaturateOnIntegerOverflow=on
  Richtung : MATLAB Function  TreatAsAtomicUnit=on  SystemSampleTime=0.01
  Sum : Sum  Inputs=|-+  SampleTime=0.01
  Verstaerkung : Gain  Gain=100  SampleTime=0.01
  pwm_out : Outport  VectorParamsAs1DForOutWhenUnconnected=off
  r/l_out : Outport  Port=2  VectorParamsAs1DForOutWhenUnconnected=off
  wires:
  Betrag/1(y) -> pwm_out/1
  Verstaerkung/1 -> Abs/1, Richtung/1(u)
  Sum/1 -> Dead Zone/1
  Abs/1 -> Begrenzung/1
  y_soll/1 -> Sum/2
  Richtung/1(y) -> r/l_out/1
  y_ist/1 -> Sum/1
  Begrenzung/1 -> Betrag/1(u)
  Dead Zone/1 -> Verstaerkung/1

== system Gesamtsystem_Prototyp25_01_3/Sortierung/Weiche/Subsystem ==
  In1 : Inport
  2 : Constant  Value=0
  3 : Constant
  Switch1 : Switch  Criteria=u2 > Threshold  Threshold=0.5
  Out1 : Outport
  wires:
  In1/1 -> Switch1/2
  3/1 -> Switch1/3
  2/1 -> Switch1/1
  Switch1/1 -> Out1/1

== system Gesamtsystem_Prototyp25_01_3/Sortierung/Weiche/Subsystem1 ==
  In1 : Inport
  0 : Constant  Value=0
  1 : Constant
  Switch : Switch  Criteria=u2 > Threshold  Threshold=0.5
  Out1 : Outport
  wires:
  1/1 -> Switch/3
  0/1 -> Switch/1
  In1/1 -> Switch/2
  Switch/1 -> Out1/1

== system Gesamtsystem_Prototyp25_01_3/Kommunikation/I2C Receiver/DecodeNexonar/Subsystem ==
  packed : Inport
  Bit Shift : hdlsllib/Logic and Bit Operations/Bit Shift  mode=Shift Left Logical  N=8
  Data Type Conversion : DataTypeConversion  OutDataTypeStr=int16
  Demux : Demux  Outputs=2
  Sum : Sum  Inputs=|++
  unpacked : Outport
  wires:
  packed/1 -> Demux/1
  Sum/1 -> Data Type Conversion/1
  Demux/1 -> Bit Shift/1
  Bit Shift/1 -> Sum/1
  Demux/2 -> Sum/2
  Data Type Conversion/1 -> unpacked/1

== system Gesamtsystem_Prototyp25_01_3/Kommunikation/I2C Receiver/DecodeNexonar/Subsystem1 ==
  packed : Inport
  Bit Shift : hdlsllib/Logic and Bit Operations/Bit Shift  mode=Shift Left Logical  N=8
  Data Type Conversion : DataTypeConversion  OutDataTypeStr=int16
  Demux : Demux  Outputs=2
  Sum : Sum  Inputs=|++
  unpacked : Outport
  wires:
  Data Type Conversion/1 -> unpacked/1
  Demux/2 -> Sum/2
  Bit Shift/1 -> Sum/1
  Demux/1 -> Bit Shift/1
  Sum/1 -> Data Type Conversion/1
  packed/1 -> Demux/1
